simulink model "MyEd_project"  (R2019a)
settings: Solver=VariableStepAuto  StartTime=0.0  StopTime=4  RelTol=1e-3
libraries: powerlib x12, simulink x2
settings Model: Creator=Arun Nair  LastModifiedBy=Arun Nair

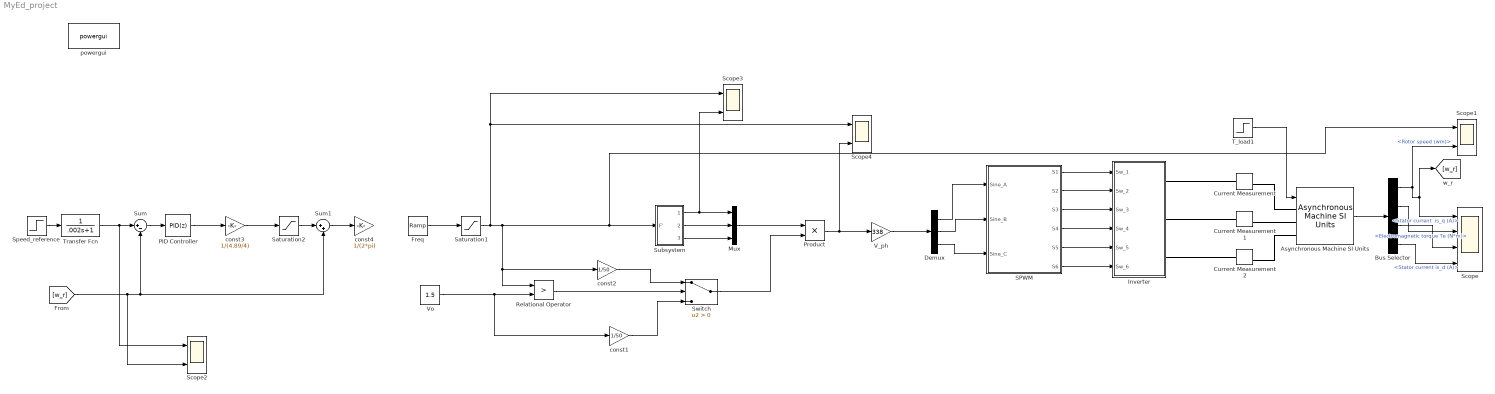
== system MyEd_project ==
  Asynchronous Machine SI Units : powerlib/Machines/Asynchronous Machine SI Units  RotorType=Squirrel-cage  PresetModel=No  MechanicalLoad=Torque Tm  ShowDetailedParameters=on  ReferenceFrame=Rotor  Units=SI  MeasurementBus=off  NominalParameters=[1.845e+04 415 50]  Stator=[0.5968 0.0003495]  Rotor=[0.6258 0.005473]  Cage1=[0.4155 0.002066]  Cage2=[0.4168 0.0003495]  Lm=0.0354  Mechanical=[0.05 0.005879 2]  PolePairs=2  InitialConditions=[1 0 0 0 0 0 0 0]  SimulateSaturation=off  Saturation=[14.03593122, 27.81365428, 53.79336849, 72.68890987, 97.98006896, 148.6815601, 215.7428561, 302.9841135, 428.7778367 ; 230, 322, 414, 460, 506, 552, 598, 644, 690]  LoadFlowParameters=1492000  TsPowergui=0  TsBlock=-1  IterativeModel=Trapezoidal non iterative  IterativeDiscreteModel=Trapezoidal non iterative  Pmec=1.492e+006
      settings: SourceProductName=Simscape Electrical
  Bus Selector : BusSelector  OutputSignals="Mechanical.Rotor speed (wm),Mechanical.Electromagnetic torque Te (N*m),Stator measurements.Stator current  is_q (A),Stator measurements.Stator current is_d (A)"
  Current Measurement : powerlib/Measurements/Current Measurement  PhasorSimulation=off  OutputType=Complex  PSBequivalent=0
      settings: SourceProductName=Simscape Electrical
  Current Measurement1 : powerlib/Measurements/Current Measurement  PhasorSimulation=off  OutputType=Complex  PSBequivalent=0
      settings: SourceProductName=Simscape Electrical
  Current Measurement2 : powerlib/Measurements/Current Measurement  PhasorSimulation=off  OutputType=Complex  PSBequivalent=0
      settings: SourceProductName=Simscape Electrical
  Demux : Demux  Outputs=3
  Freq : simulink/Sources/Ramp  slope=50  start=0  InitialOutput=0
  Inverter : Subsystem
  Mux : Mux  Inputs=3
  PID Controller : simulink/Continuous/PID Controller  Controller=PID  Form=Parallel  TimeDomain=Discrete-time  SampleTime=-1  IntegratorMethod=Forward Euler  FilterMethod=Forward Euler  ControllerParametersSource=internal  P=0.0930*1000  I=0.0000001  D=0  UseFilter=on  N=100  TunerSelectOption=Transfer Function Based (PID Tuner App)  InitialConditionSource=internal  InitialConditionForIntegrator=0  InitialConditionForFilter=0  DifferentiatorICPrevScaledInput=0  ExternalReset=none  TrackingMode=off  Kt=1  LimitOutput=off  UpperSaturationLimit=inf  LowerSaturationLimit=-inf  LinearizeAsGain=on  AntiWindupMode=none  Kb=1  POutMin=[]  POutMax=[]  IOutMin=[]  IOutMax=[]  DOutMin=[]  DOutMax=[]  NOutMin=[]  NOutMax=[]  SumOutMin=[]  SumOutMax=[]  SaturationOutMin=[]  SaturationOutMax=[]  PParamMin=[]  PParamMax=[]  IParamMin=[]  IParamMax=[]  DParamMin=[]  DParamMax=[]  NParamMin=[]  NParamMax=[]  KbParamMin=[]  KbParamMax=[]  KtParamMin=[]  KtParamMax=[]  KbOutMin=[]  KbOutMax=[]  KtOutMin=[]  KtOutMax=[]  IntegratorOutMin=[]  IntegratorOutMax=[]  FilterOutMin=[]  FilterOutMax=[]  SumI1OutMin=[]  SumI1OutMax=[]  SumI2OutMin=[]  SumI2OutMax=[]  SumI3OutMin=[]  SumI3OutMax=[]  SumI4OutMin=[]  SumI4OutMax=[]  SumDOutMin=[]  SumDOutMax=[]  DifferentiatorOutMin=[]  DifferentiatorOutMax=[]  FilterDiffOutCoefMin=[]  FilterDiffOutCoefMax=[]  ReciprocalOutMin=[]  ReciprocalOutMax=[]  SumDenOutMin=[]  SumDenOutMax=[]  SumNumOutMin=[]  SumNumOutMax=[]  DivideOutMin=[]  DivideOutMax=[]  IntegratorContinuousStateAttributes=''  IntegratorStateMustResolveToSignalObject=off  IntegratorRTWStateStorageClass=Auto  FilterContinuousStateAttributes=''  FilterStateMustResolveToSignalObject=off  FilterRTWStateStorageClass=Auto  ParallelPVariant=InternalParameters  IdealPVariant=Disabled  IVariant=InternalParameters  DVariant=InternalParameters  IntegratorVariant=Discrete  SatVariant=Disabled  AWVariant=Passthrough  PCopyVariant=Disabled  TRVariant=Disabled  FdbkBlocksVariant=Forward  IdealPFdbkVariant=Disabled  SatFdbkVariant=Disabled  DerivativeFilterVariant=ForwardEulerFilter  NVariant=InternalParameters  NCopyVariant=Disabled  FilterICVariant=InternalICsFilter  IntegratorICVariant=InternalICs  ExternalResetVariant=Disabled  TRSumVariant=Passthrough  SumFdbkVariant=Disabled  SumVariant=Sum_PID
  Product : Product
  Relational Operator : RelationalOperator  Operator=>  OutDataTypeStr=boolean  RndMeth=Simplest
  SPWM : Subsystem
  Saturation1 : Saturate  UpperLimit=50  LowerLimit=0
  Saturation2 : Saturate  UpperLimit=377  LowerLimit=-377
  Scope : Scope  NumInputPorts=4
  Scope{1..4} (4 alike) : Scope  NumInputPorts=2
  Speed_reference : Step  Time=0.6  Before=50  After=150
  Subsystem : Subsystem
  Sum : Sum  Inputs=|+-
  Sum1 : Sum  Inputs=|++
  Switch : Switch  Criteria=u2 > Threshold
  T_load1 : Step  Time=10  Before=20  After=5
  Transfer Fcn : TransferFcn  Denominator=[.002 1]
  V_ph : Gain  Gain=338
  Vo : Constant  Value=1.5
  const1 : Gain  Gain=1/50
  const2 : Gain  Gain=1/50
  const3 : Gain  Gain=1/(4.89/4)
  const4 : Gain  Gain=1/(2*pi)
  "powergui " : powerlib/powergui  Priority=1  SimulationMode=Discrete  SampleTime=1e-6  frequency=60  Iterations=50  frequencyindice=50  Pbase=100e6  ErrMax=1e-4  UnitsV=kV  UnitsW=MW  buscounter=0  FunctionMessages=off  echomessages=off  EnableUseOfTLC=off  CurrentSourceSwitches=off  DisableSnubberDevices=off  DisableRonSwitches=off  DisableVfSwitches=off  DisplayEquations=off  AutomaticDiscreteSolvers=off  SolverType=Tustin/Backward Euler (TBE)  Interpol=off  ExternalGateDelay=off  methode=off  Ts=100  x0status=blocks  SPID=on  SwTol=0  HookPort=off  NonlinearTolerance=0  nMaxIteration=15  ContinueOnMaxIteration=off  RestoreLinks=warning  ResistiveCurrentMeasurement=off  Frange=[0:2:500]  Ylog=off  Xlog=on  ShowGrid=off  save=off  variable=ZData  structure=0  ZoomFFT=off  StartTime=0.0  cycles=1  DisplayStyle=1  fundamental=60  FreqAxis=off  MaxFrequency=1000  frequencyindicesteady=1  RmsSteady=1  display=off
      settings: SourceProductName=Simscape Electrical
  wires:
  SPWM/1(S1) -> Inverter/1(Sw_1)
  Sum1/1 -> const4/1
  Transfer Fcn/1 -> Scope2/1, Sum/1
  T_load1/1 -> Asynchronous Machine SI Units/1
  SPWM/6(S6) -> Inverter/6(Sw_6)
  Demux/3 -> SPWM/3(Sine_C)
  Saturation2/1 -> Sum1/1
  const3/1 -> Saturation2/1
  Bus Selector/2 -> Scope/2  "<Electromagnetic torque Te (N*m)>"
  Subsystem/3(SinC) -> Mux/3
  PID Controller/1 -> const3/1
  [w_r] -> Scope2/2, Sum1/2, Sum/2
  Product/1 -> Scope4/2, V_ph/1
  Sum/1 -> PID Controller/1
  Speed_reference/1 -> Transfer Fcn/1
  Bus Selector/1 -> [w_r], Scope/1, Scope1/2  "<Rotor speed (wm)>"
  Asynchronous Machine SI Units/1 -> Bus Selector/1
  Demux/2 -> SPWM/2(Sine_B)
  SPWM/5(S5) -> Inverter/5(Sw_5)
  SPWM/4(S4) -> Inverter/4(Sw_4)
  Demux/1 -> SPWM/1(Sine_A)
  Subsystem/2(SinB) -> Mux/2
  SPWM/3(S3) -> Inverter/3(Sw_3)
  Saturation1/1 -> Scope4/1, Scope3/1, Scope1/1, Subsystem/1(F'), Relational Operator/1, const2/1
  SPWM/2(S2) -> Inverter/2(Sw_2)
  const1/1 -> Switch/3
  V_ph/1 -> Demux/1
  const2/1 -> Switch/1
  Relational Operator/1 -> Switch/2
  Vo/1 -> const1/1, Relational Operator/2
  Mux/1 -> Product/1
  Switch/1 -> Product/2
  Subsystem/1(SinA) -> Scope3/2, Mux/1
  Freq/1 -> Saturation1/1
  Bus Selector/3 -> Scope/3  "<Stator current  is_q (A)>"
  Bus Selector/4 -> Scope/4  "<Stator current is_d (A)>"
  connections:
  Current Measurement2/RConn1 -- Asynchronous Machine SI Units/LConn3
  Current Measurement/LConn1 -- Inverter/RConn1
  Current Measurement1/RConn1 -- Asynchronous Machine SI Units/LConn2
  Current Measurement1/LConn1 -- Inverter/RConn2
  Current Measurement/RConn1 -- Asynchronous Machine SI Units/LConn1
  Current Measurement2/LConn1 -- Inverter/RConn3

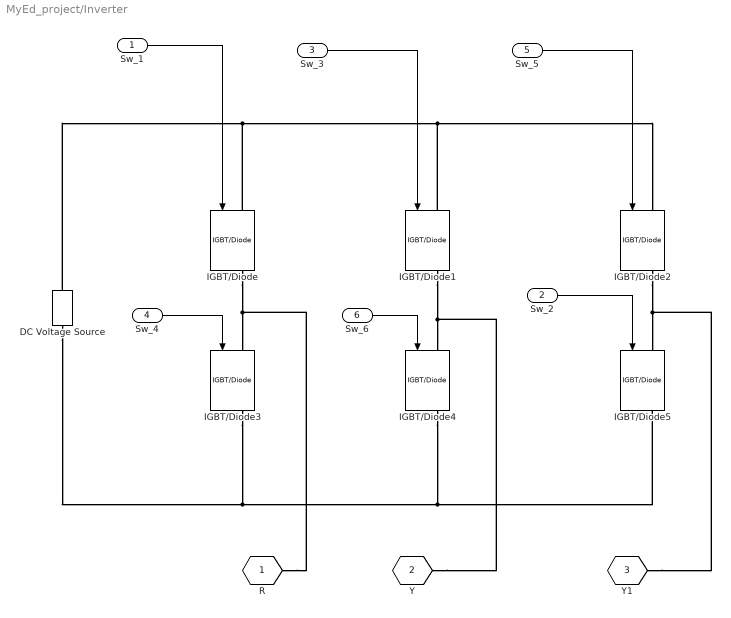
== system MyEd_project/Inverter ==
  Sw_1 : Inport
  Sw_2 : Inport  Port=2
  Sw_3 : Inport  Port=3
  Sw_4 : Inport  Port=4
  Sw_5 : Inport  Port=5
  Sw_6 : Inport  Port=6
  DC Voltage Source : powerlib/Electrical Sources/DC Voltage Source  Amplitude=700  Measurements=None
      settings: SourceProductName=Simscape Electrical
  IGBT/Diode{,1..5} (6 alike) : powerlib/Power Electronics/IGBT//Diode  Ron=1e-3  Rs=1e5  Cs=inf  Measurements=on
      settings: SourceProductName=Simscape Electrical
  R : PMIOPort  Tag=PMCPort  Side=Right
  Y : PMIOPort  Tag=PMCPort  Port=2  Side=Right
  Y1 : PMIOPort  Tag=PMCPort  Port=3  Side=Right
  wires:
  Sw_4/1 -> IGBT/Diode3/1
  Sw_3/1 -> IGBT/Diode1/1
  Sw_2/1 -> IGBT/Diode5/1
  Sw_1/1 -> IGBT/Diode/1
  Sw_6/1 -> IGBT/Diode4/1
  Sw_5/1 -> IGBT/Diode2/1
  connections:
  DC Voltage Source/RConn1 -- IGBT/Diode/LConn1 -- IGBT/Diode1/LConn1 -- IGBT/Diode2/LConn1
  DC Voltage Source/LConn1 -- IGBT/Diode3/RConn1 -- IGBT/Diode4/RConn1 -- IGBT/Diode5/RConn1
  IGBT/Diode1/RConn1 -- Y/RConn1 -- IGBT/Diode4/LConn1
  IGBT/Diode2/RConn1 -- Y1/RConn1 -- IGBT/Diode5/LConn1
  IGBT/Diode/RConn1 -- R/RConn1 -- IGBT/Diode3/LConn1

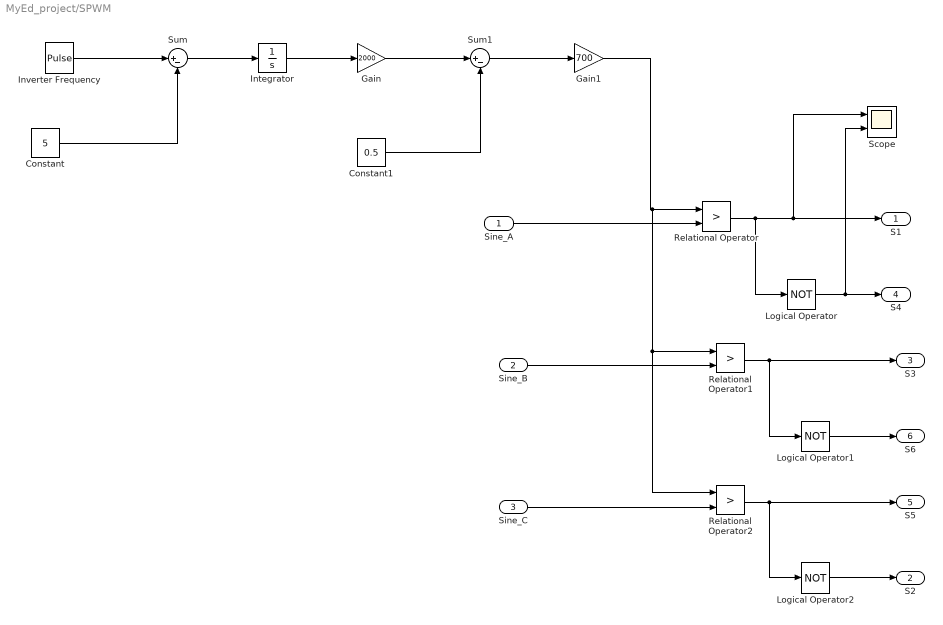
== system MyEd_project/SPWM ==
  Sine_A : Inport
  Sine_B : Inport  Port=2
  Sine_C : Inport  Port=3
  Constant : Constant  Value=5
  Constant1 : Constant  Value=0.5
  Gain : Gain  Gain=2000
  Gain1 : Gain  Gain=700
  Integrator : Integrator
  Inverter Frequency : DiscretePulseGenerator  PulseType=Time based  Amplitude=10  Period=2e-4  PulseWidth=50
  Logical Operator : Logic  Operator=NOT  AllPortsSameDT=off  OutDataTypeStr=boolean
  Logical Operator1 : Logic  Operator=NOT  AllPortsSameDT=off  OutDataTypeStr=boolean
  Logical Operator2 : Logic  Operator=NOT  AllPortsSameDT=off  OutDataTypeStr=boolean
  Relational Operator : RelationalOperator  Operator=>  OutDataTypeStr=boolean  RndMeth=Simplest
  Relational Operator1 : RelationalOperator  Operator=>  OutDataTypeStr=boolean  RndMeth=Simplest
  Relational Operator2 : RelationalOperator  Operator=>  OutDataTypeStr=boolean  RndMeth=Simplest
  Scope : Scope  NumInputPorts=2
  Sum : Sum  Inputs=|+-
  Sum1 : Sum  Inputs=|+-
  S1 : Outport
  S2 : Outport  Port=2
  S3 : Outport  Port=3
  S4 : Outport  Port=4
  S5 : Outport  Port=5
  S6 : Outport  Port=6
  wires:
  Sine_B/1 -> Relational Operator1/2
  Gain/1 -> Sum1/1
  Relational Operator/1 -> Scope/1, S1/1, Logical Operator/1
  Relational Operator1/1 -> S3/1, Logical Operator1/1
  Sum1/1 -> Gain1/1
  Logical Operator1/1 -> S6/1
  Inverter Frequency/1 -> Sum/1
  Gain1/1 -> Relational Operator2/1, Relational Operator1/1, Relational Operator/1
  Constant1/1 -> Sum1/2
  Sum/1 -> Integrator/1
  Constant/1 -> Sum/2
  Integrator/1 -> Gain/1
  Sine_A/1 -> Relational Operator/2
  Logical Operator/1 -> Scope/2, S4/1
  Logical Operator2/1 -> S2/1
  Sine_C/1 -> Relational Operator2/2
  Relational Operator2/1 -> S5/1, Logical Operator2/1

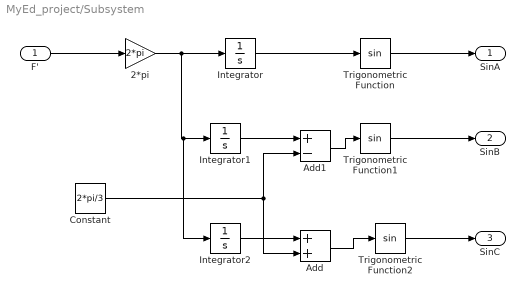
== system MyEd_project/Subsystem ==
  F' : Inport
  2*pi : Gain  Gain=2*pi
  Add : Sum
  Add1 : Sum  Inputs=+-
  Constant : Constant  Value=2*pi/3
  Integrator : Integrator
  Integrator1 : Integrator
  Integrator2 : Integrator
  Trigonometric Function : Trigonometry
  Trigonometric Function1 : Trigonometry
  Trigonometric Function2 : Trigonometry
  SinA : Outport
  SinB : Outport  Port=2
  SinC : Outport  Port=3
  wires:
  Integrator2/1 -> Add/1
  Trigonometric Function/1 -> SinA/1
  Trigonometric Function2/1 -> SinC/1
  Trigonometric Function1/1 -> SinB/1
  2*pi/1 -> Integrator2/1, Integrator1/1, Integrator/1
  Constant/1 -> Add1/2, Add/2
  Integrator1/1 -> Add1/1
  Integrator/1 -> Trigonometric Function/1
  F'/1 -> 2*pi/1
  Add/1 -> Trigonometric Function2/1
  Add1/1 -> Trigonometric Function1/1
